simulink model "part1"  (R2019b)
settings: Solver=VariableStepAuto  StartTime=0.0  StopTime=1800  RelTol=1e-3
values from neighbouring files (symbols this model uses):
  corner_test = 1    [pick_sp.m]
  corners = [0,0,0;50,0,0;50,-50,0;50,-50,-pi/4;0,-50,-pi/4;0,0,0]    [pick_sp.m]
  curr_const = 1    [pick_sp.m]
  curr_vel = 0    [pick_sp.m]
  Kd = [1e+07,1e+07,2e+08]    [tune.m]
  Ki = [1e+02,3e+03,1e+02]    [tune.m]
  Kp = [5e+05,5e+05,2e+07]    [tune.m]
  ref_model_on = 1    [pick_sp.m]
  setpoint = [10,10,1.5*pi]    [pick_sp.m]
  w_n = [0.08,0.04,0.03]    [tune.m]
  zeta = 1    [tune.m]
undefined symbols (not defined in the file or in its folder): Hoerner, vessel
libraries: marine_gnc x7, simulink x1, marine_hydro x1
settings Model: Creator=jonbjor  LastModifiedBy=Elias
settings DataIOCC: ReturnWorkspaceOutputs=off
settings DebuggingCC: ArithmeticOperatorsInVariantConditions=warning
settings SFSimCC: SimUseLocalCustomCode=off  CustomCodeUndefinedFunction=UseInterfaceOnly
settings RTWCC: RTWUseLocalCustomCode=off

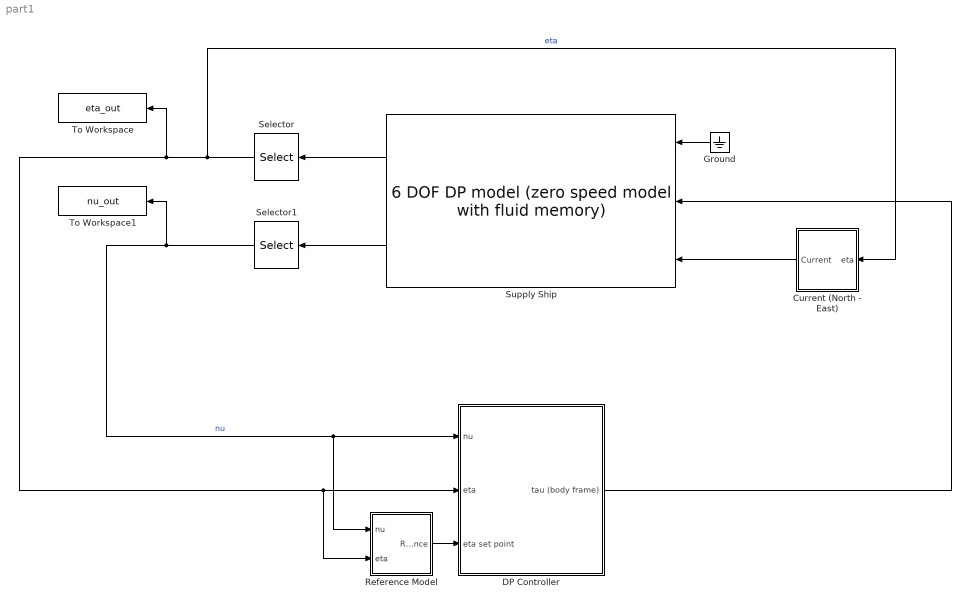
== system part1 ==
  Current (North - East) : Subsystem
  DP Controller : Subsystem
  Ground : Ground
  Reference Model : Subsystem
  Selector : Selector  InputPortWidth=6  IndexOptions=Index vector (dialog)  Indices=[1 2 6]  OutputSizes=1
  Selector1 : Selector  InputPortWidth=6  IndexOptions=Index vector (dialog)  Indices=[1 2 6]  OutputSizes=1
  Supply Ship : marine_hydro/Hydro Library/6 DOF DP model  (zero speed model with fluid memory)  ABC=vesselABC  rho=1025  Axc=0.9*vessel.main.T*vessel.main.B  Ayc=0.9*vessel.main.T*vessel.main.Lpp  CX=1  CY_2D=Hoerner(vessel.main.B,vessel.main.T)  Bv=vessel.Bv  mask(6 DOF zero speed model){}
      link override "Integrator1 ": InitialCondition=nu0
      link override Integrator2: InitialCondition=eta0
      settings: SourceProductName=MSS Hydro
      mask Display:
      | image('supply.jpg');
      | color('white'); port_label('output', 1, 'eta')
      | color('white'); port_label('output', 2, 'nu')
      | color('white'); port_label('input', 1, 'tau_wave')
      | color('white'); port_label('input', 2, 'tau')
      | color('white'); port_label('input', 3, 'nu_c')
  To Workspace : ToWorkspace  VariableName=eta_out  SampleTime=-1
  To Workspace1 : ToWorkspace  VariableName=nu_out  SampleTime=-1
  wires:
  DP Controller/1(tau (body frame)) -> Supply Ship/2
  Supply Ship/1 -> Selector/1
  Supply Ship/2 -> Selector1/1
  Reference Model/1("Reference ") -> DP Controller/3(eta set point)
  Selector/1 -> Current (North - East)/1(eta), Reference Model/2(eta), DP Controller/2(eta), To Workspace/1  "eta"
  Selector1/1 -> To Workspace1/1, Reference Model/1(nu), DP Controller/1(nu)  "nu"
  Current (North - East)/1(Current) -> Supply Ship/3
  Ground/1 -> Supply Ship/1

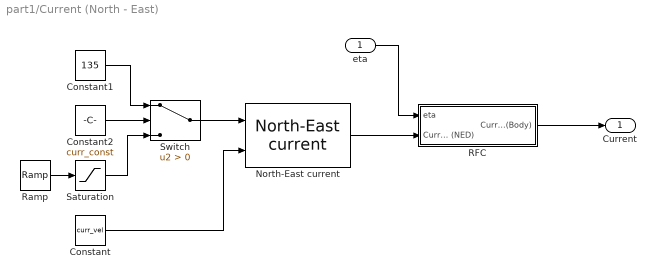
== system part1/Current (North - East) ==
  eta : Inport
  Constant : Constant  Value=curr_vel
  Constant1 : Constant  Value=135
  Constant2 : Constant  Value=curr_const
  North-East current : marine_gnc/Environment/Current/North-East current  SystemSampleTime=-1  Latency=0  AutoFrameSizeCalculation=off
      settings: SourceProductName=MSS GNC
  "RFC " : Subsystem
  Ramp : simulink/Sources/Ramp  slope=90/300  start=0  InitialOutput=180
  Saturation : Saturate  UpperLimit=270
  Switch : Switch  Criteria=u2 > Threshold
  Current : Outport  VectorParamsAs1DForOutWhenUnconnected=off
  wires:
  North-East current/1 -> "RFC "/2("Current (NED) ")
  Constant1/1 -> Switch/1
  Constant/1 -> North-East current/2
  "RFC "/1("Current (Body) ") -> Current/1
  eta/1 -> "RFC "/1(eta)
  Switch/1 -> North-East current/1
  Saturation/1 -> Switch/3
  Constant2/1 -> Switch/2
  Ramp/1 -> Saturation/1

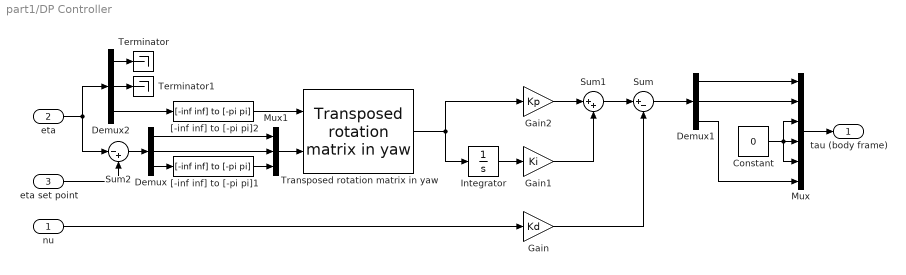
== system part1/DP Controller ==
  nu : Inport  PortDimensions=3
  eta : Inport  Port=2  PortDimensions=3
  eta set point : Inport  Port=3
  Constant : Constant  Value=0
  Demux : Demux  Outputs=3
  Demux1 : Demux  Outputs=3
  Demux2 : Demux  Outputs=3
  Gain : Gain  Gain=Kd
  Gain1 : Gain  Gain=Ki
  Gain2 : Gain  Gain=Kp
  Integrator : Integrator
  Mux : Mux  Inputs=6
  Mux1 : Mux  Inputs=3
  Sum : Sum  Inputs=|+-
  Sum1 : Sum  Inputs=|++
  Sum2 : Sum  Inputs=|-+
  Terminator : Terminator
  Terminator1 : Terminator
  Transposed rotation matrix in yaw : marine_gnc/Models/ Kinematics/Transposed rotation  matrix in yaw
      settings: SourceProductName=MSS GNC
  "[-inf inf] to [-pi pi]1" : marine_gnc/Utilities/Math Operations/[-inf inf] to [-pi pi]
      settings: SourceProductName=MSS GNC
  "[-inf inf] to [-pi pi]2" : marine_gnc/Utilities/Math Operations/[-inf inf] to [-pi pi]
      settings: SourceProductName=MSS GNC
  tau (body frame) : Outport  VectorParamsAs1DForOutWhenUnconnected=off
  wires:
  eta set point/1 -> Sum2/2
  nu/1 -> Gain/1
  eta/1 -> Demux2/1, Sum2/1
  Sum/1 -> Demux1/1
  Gain/1 -> Sum/2
  Sum1/1 -> Sum/1
  Integrator/1 -> Gain1/1
  Gain1/1 -> Sum1/2
  Gain2/1 -> Sum1/1
  Transposed rotation matrix in yaw/1 -> Integrator/1, Gain2/1
  Demux2/3 -> "[-inf inf] to [-pi pi]2"/1
  Demux2/2 -> Terminator1/1
  Demux2/1 -> Terminator/1
  "[-inf inf] to [-pi pi]2"/1 -> Transposed rotation matrix in yaw/1
  Sum2/1 -> Demux/1
  Demux/1 -> Mux1/1
  Demux/2 -> Mux1/2
  Demux/3 -> "[-inf inf] to [-pi pi]1"/1
  "[-inf inf] to [-pi pi]1"/1 -> Mux1/3
  Mux1/1 -> Transposed rotation matrix in yaw/2
  Mux/1 -> tau (body frame)/1
  Constant/1 -> Mux/5, Mux/3, Mux/4
  Demux1/2 -> Mux/2
  Demux1/1 -> Mux/1
  Demux1/3 -> Mux/6

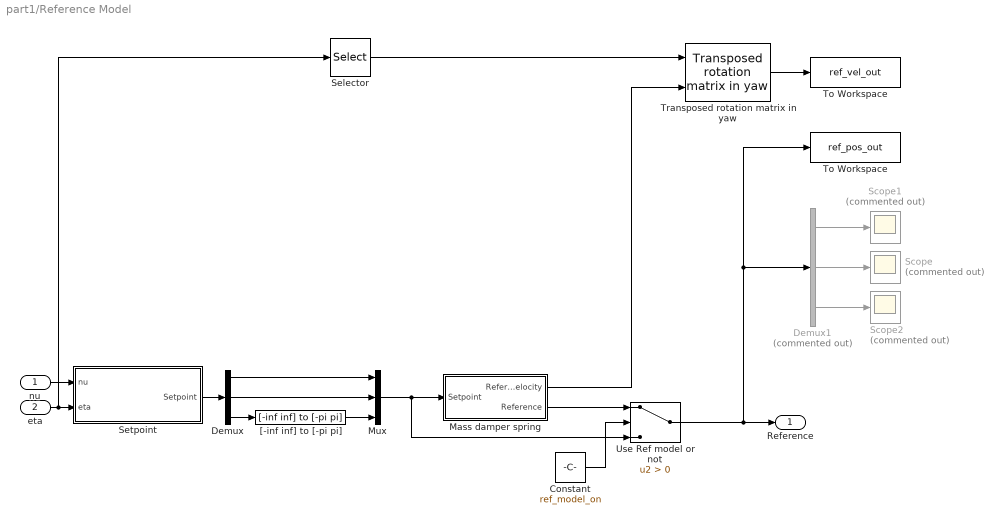
== system part1/Reference Model ==
  nu : Inport
  eta : Inport  Port=2
  Constant : Constant  Value=ref_model_on
  Demux : Demux  Outputs=3
  Demux1 : Demux  Commented=on  Outputs=3
  Mass damper spring : Subsystem
  Mux : Mux  Inputs=3
  Scope : Scope  Commented=on
  Scope1 : Scope  Commented=on
  Scope2 : Scope  Commented=on
  Selector : Selector  InputPortWidth=3  IndexOptions=Index vector (dialog)  Indices=[3]  OutputSizes=1
  "Setpoint " : Subsystem
  To Workspace : ToWorkspace  VariableName=ref_vel_out  SampleTime=-1
  "To Workspace " : ToWorkspace  VariableName=ref_pos_out  SampleTime=-1
  Transposed rotation matrix in yaw : marine_gnc/Models/ Kinematics/Transposed rotation  matrix in yaw
      settings: SourceProductName=MSS GNC
  Use Ref model or not : Switch  Criteria=u2 > Threshold
  "[-inf inf] to [-pi pi]" : marine_gnc/Utilities/Math Operations/[-inf inf] to [-pi pi]
      settings: SourceProductName=MSS GNC
  "Reference " : Outport  VectorParamsAs1DForOutWhenUnconnected=off
  wires:
  Demux/1 -> Mux/1
  Demux/2 -> Mux/2
  Demux/3 -> "[-inf inf] to [-pi pi]"/1
  "[-inf inf] to [-pi pi]"/1 -> Mux/3
  "Setpoint "/1("Setpoint ") -> Demux/1
  nu/1 -> "Setpoint "/1(nu)
  Demux1/2 -> Scope/1
  Demux1/1 -> Scope1/1
  Demux1/3 -> Scope2/1
  Mux/1 -> Use Ref model or not/3, Mass damper spring/1("Setpoint ")
  Mass damper spring/2("Reference ") -> Use Ref model or not/1
  Constant/1 -> Use Ref model or not/2
  Mass damper spring/1("Reference Velocity ") -> Transposed rotation matrix in yaw/2
  Transposed rotation matrix in yaw/1 -> To Workspace/1
  eta/1 -> Selector/1, "Setpoint "/2("eta ")
  Use Ref model or not/1 -> "To Workspace "/1, Demux1/1, "Reference "/1
  Selector/1 -> Transposed rotation matrix in yaw/1

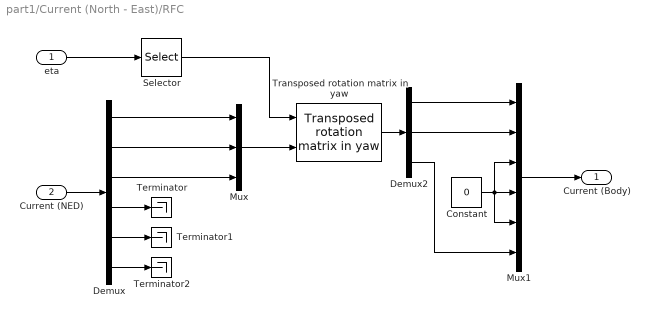
== system part1/Current (North - East)/RFC  ==
  eta : Inport
  "Current (NED) " : Inport  Port=2
  Constant : Constant  Value=0
  Demux : Demux  Outputs=6
  Demux2 : Demux  Outputs=3
  Mux : Mux  Inputs=3
  Mux1 : Mux  Inputs=6
  Selector : Selector  InputPortWidth=3  IndexOptions=Index vector (dialog)  Indices=[3]  OutputSizes=1
  Terminator : Terminator
  Terminator1 : Terminator
  Terminator2 : Terminator
  Transposed rotation matrix in yaw : marine_gnc/Models/ Kinematics/Transposed rotation  matrix in yaw
      settings: SourceProductName=MSS GNC
  "Current (Body) " : Outport
  wires:
  eta/1 -> Selector/1
  Selector/1 -> Transposed rotation matrix in yaw/1
  Demux/3 -> Mux/3
  Demux/2 -> Mux/2
  Demux/1 -> Mux/1
  Mux/1 -> Transposed rotation matrix in yaw/2
  Mux1/1 -> "Current (Body) "/1
  Transposed rotation matrix in yaw/1 -> Demux2/1
  Demux2/3 -> Mux1/6
  Demux2/1 -> Mux1/1
  Constant/1 -> Mux1/5, Mux1/3, Mux1/4
  "Current (NED) "/1 -> Demux/1
  Demux/4 -> Terminator/1
  Demux/5 -> Terminator1/1
  Demux/6 -> Terminator2/1
  Demux2/2 -> Mux1/2

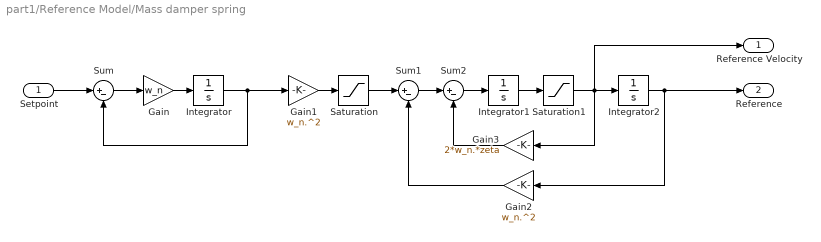
== system part1/Reference Model/Mass damper spring ==
  "Setpoint " : Inport
  Gain : Gain  Gain=w_n
  Gain1 : Gain  Gain=w_n.^2
  Gain2 : Gain  Gain=w_n.^2
  Gain3 : Gain  Gain=2*w_n.*zeta
  Integrator : Integrator
  Integrator1 : Integrator
  Integrator2 : Integrator
  Saturation : Saturate  UpperLimit=25  LowerLimit=-25
  Saturation1 : Saturate  UpperLimit=25  LowerLimit=-25
  Sum : Sum  Inputs=|+-
  Sum1 : Sum  Inputs=|+-
  Sum2 : Sum  Inputs=|+-
  "Reference Velocity " : Outport
  "Reference " : Outport  Port=2
  wires:
  Gain1/1 -> Saturation/1
  Saturation/1 -> Sum1/1
  Saturation1/1 -> "Reference Velocity "/1, Gain3/1, Integrator2/1
  Gain/1 -> Integrator/1
  Sum2/1 -> Integrator1/1
  Integrator1/1 -> Saturation1/1
  Sum1/1 -> Sum2/1
  Gain3/1 -> Sum2/2
  Integrator/1 -> Gain1/1, Sum/2
  Integrator2/1 -> "Reference "/1, Gain2/1
  Sum/1 -> Gain/1
  Gain2/1 -> Sum1/2
  "Setpoint "/1 -> Sum/1

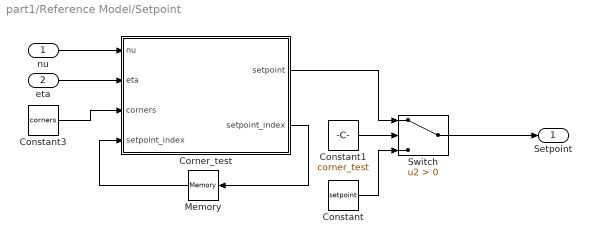
== system part1/Reference Model/Setpoint  ==
  nu : Inport
  "eta " : Inport  Port=2
  Constant : Constant  Value=setpoint
  Constant1 : Constant  Value=corner_test
  Constant3 : Constant  Value=corners
  Corner_test : MATLAB Function  TreatAsAtomicUnit=on
  Memory : Memory  InitialCondition=1
  Switch : Switch  Criteria=u2 > Threshold
  "Setpoint " : Outport
  wires:
  Constant/1 -> Switch/3
  Switch/1 -> "Setpoint "/1
  Constant1/1 -> Switch/2
  Corner_test/1(setpoint) -> Switch/1
  "eta "/1 -> Corner_test/2(eta)
  nu/1 -> Corner_test/1(nu)
  Constant3/1 -> Corner_test/3(corners)
  Corner_test/2(setpoint_index) -> Memory/1
  Memory/1 -> Corner_test/4("setpoint_index ")

== matlab function part1/Reference Model/Setpoint /Corner_test ==
  data: nu input; eta input; corners input; setpoint output; setpoint_index input; setpoint_index output
function [setpoint,setpoint_index] = fcn(nu, eta, corners, setpoint_index)

setpoint=corners(setpoint_index,:);

eta_tol = [0.5,0.5,pi/180];
nu_tol = [0.05,0.05,0.01];

err = [abs(setpoint-eta');abs(nu')];
test = err > [eta_tol;nu_tol];

if (sum(sum(test)) == 0)
    setpoint_index = mod(setpoint_index,6)+1;
    % NB: The corner test will loop once finished.
end
